simulink model "husky_sim"  (R2019b)
settings: Solver=ode4  StartTime=0.0  StopTime=8  FixedStep=Ts  RelTol=1e-3
InitFcn:
  | init_model;
values from neighbouring files (symbols this model uses):
  backbone_mass_pos_wrt_body = [0.021107, -5.5457e-05, -0.041523]    [func_robot_param.m]
  del_p_FL_1 = [0.0, 0.18, 0.1]    [func_params_ext.m]
  del_p_FL_2 = [0.0, 0, 0.15]    [func_params_ext.m]
  del_y_BL = 0.125/n    (= 0.0125)    [func_params_ext.m]
  del_y_BR = 0.125/n    (= 0.0125)    [func_params_ext.m]
  del_z_BL = z_BL(2:end)-z_BL(1:n)    [func_params_ext.m]
  del_z_BR = z_BR(2:end)-z_BR(1:n)    [func_params_ext.m]
  femur_mass_loc = [2.704e-07, -0.036112, -0.082829]    [func_params_ext.m]    (also in func_robot_param.m)
  hip_orgin_wrt_backbone = [hip_FR_origin_wrt_backbone, hip_FL_origin_wrt_backbone, hip_BR_origin_wrt_backbone, hip_BL_origin_wrt_backbone].'    [func_params_ext.m]    (also in func_robot_param.m)
  leg_params = [l_hip_offset, l1, l2, l3, q_hf_offset, q_hs_offset, q_k_offset]    [func_params_ext.m]
  m = getfield(leg,'mass')    [dynamic_test.m]    (also in pen_init.m = link2.mass; test.mat = 2.2337)
  mu_s = 0.8    [func_params_ext.m]    (also in pen_init.m; test.mat)
  n = 10    [func_params_ext.m]
  p_init = p_init + 1*[0,0,0,  0,0,0,  0,-0,0,   0,0,0]    [func_params_ext.m]
  q_BL_K0 = initial_angle(12)    [func_params_ext.m]
  q_BR_K0 = initial_angle(9)    [func_params_ext.m]
  q_FL_K0 = initial_angle(6)    [func_params_ext.m]
  T_f_back_BL = 0.1/n    (= 0.01)    [func_params_ext.m]
  T_f_back_BR = 0.1/n    (= 0.01)    [func_params_ext.m]
  T_f_FL_1 = 1    [func_params_ext.m]
  T_f_FL_2 = 1    [func_params_ext.m]
  t_start = 0.32    [func_params_ext.m]
  Ts = 0.001    [func_params_ext.m]
  v_y = 0    [func_params_ext.m]
  v_z = 0    [func_params_ext.m]
undefined symbols (not defined in the file or in its folder): body, femur_left, femur_right, hip_left, hip_right, link_left, link_right, tarsus_left, tarsus_right, tibia_left, tibia_right, X, Y, Z
libraries: sm_lib x206, nesl_utility x56, dspsigops x7, Contact_Forces_Lib x4, simulink x2
(part 6 of 6)

== matlab function husky_sim/move_inside_support_triangle ==
  data: q input; del_q_req output; p_leg_end_position_0 output; p_body input; quat_body input; F_n input; F_t input; start_optimizer input; legs_on_ground input; leg_params parameter; backbone_mass_pos_wrt_body parameter; body parameter; hip_orgin_wrt_backbone parameter; femur_left parameter; femur_mass_loc parameter; p_COM_0 output; p_COM_req output; inside_triangle output; mu_s parameter; t_start parameter; t input
% Find change in joint angles necessary to move COM inside support polygon
%
% Inputs: 
%   q - (12x1) all joint angles in the follwoing order
%       [q_FR_HF; q_FR_HS; q_FR_K;
%       q_FL_HF; q_FL_HS; q_FL_K
%       q_BR_HF; q_BR_HS; q_BR_K
%       q_BL_HF; q_BL_HS; q_BL_K]
%   p_body -  (3x1) body positions [x,y,z] relative to world coordinate frame
%   quat_body - (4x1) quaternion repretsentation of body orientation 
%       relative to world coordinate frame
%   F_n: (4x1) normal forces acting on all 4 legs in the following order:
%           FR, FL, BR, BL
%   F_t: (12x1) tangential forces (x,y,z(?)) acting on the 4 legs 
% 
% Prameters: 
%   leg_params - parameters needed for computing FK or IK in each leg
%       [l_hip_offset, l1, l2, l3, q_hf_offset, q_hs_offset, q_k_offset]
%       (see notes)
%   backbone_mass_pos_wrt_body - location [x,y,z] of backbone mass 
%       relative to body cooridnate frame
%   body - structure which contains mass and inertial properties of backbone
%           used to obtain body mass
%   hip_orgin_wrt_backbone - (1x12) position [x,y,z] of hip coordinate frame of
%       each leg relative to body
%   femur_left - structure which contains mass and inertial properties of
%       femur used to obtain mass of femur (same for lef and right femur)
%   femur_mass_loc - (12x1) location [x,y,z] of all 4 femur mass relative to 
%   	hip reference frame
%   mu_s: static coeff of friciton between leg end and ground
%
% Output: 
%   del_q_req - change in joint angles necessary for the COM to be inside
%       cupport polygon, as provided by optimizer
%   p_leg_end_position_0 - (12x1) leg end position relative to world
%       coordinate frame
%   p_COM_0 - current COM position [x,y,z] relative to world coordinate frame
%   p_COM_req - COM position needed to land inside support polygon as
%       computed by optimizer
%   inside_triangle - boolean, 1 if inside support polygon, 0 otherwise
%
% NOTES: 
%   *Currently this only works when 3 legs are on the ground
%   *if optimizer fails or fi currently inside support polygon, 
%           del_q_req returns zeros (12x1)
%   *Currently it is assumed that only three legs (FR, BR, BL) are on the
%   ground if even this might not be true. This is hard coded in
%   TODO: automatically detect which legs are on the ground and compute
%       required correction
%
function [del_q_req, p_leg_end_position_0, p_COM_0, p_COM_req, inside_triangle] =...
    func_move_inside_support_polygon(q, p_body, quat_body, F_n, F_t, start_optimizer, legs_on_ground,...
    leg_params, backbone_mass_pos_wrt_body, body, hip_orgin_wrt_backbone, ...
    femur_left, femur_mass_loc, mu_s, t_start, t)

leg_on_ground_index = find(legs_on_ground);
leg_in1 = (leg_on_ground_index(1)-1)*3*[1 1 1] + [1 2 3];
leg_in2 = (leg_on_ground_index(2)-1)*3*[1 1 1] + [1 2 3];
leg_in3 = (leg_on_ground_index(3)-1)*3*[1 1 1] + [1 2 3];

leg_in = [leg_in1 leg_in2 leg_in3];

leg_out = (find(~legs_on_ground)-1)*3*[1 1 1] + [1 2 3];

% turn quaternion double vector to quaternion array
quaternion_body = quaternion(quat_body.');

% Mass of femur and body
body_mass = body.mass;
femur_mass = femur_left.mass;

p_leg_end_position_0 = func_leg_end_pos(q, p_body, quaternion_body, leg_params, hip_orgin_wrt_backbone);

% Currnet p_COM
p_COM_0 = func_husky_COM(q, p_body, leg_params, femur_mass_loc, body_mass, femur_mass, hip_orgin_wrt_backbone, backbone_mass_pos_wrt_body);
% desiired p_COM
p_COM_des = [p_body(1:2); 0.39];


% Check if inside support polygon
inside_triangle = func_check_inside_polygon(p_COM_0, p_leg_end_position_0, legs_on_ground);

if inside_triangle >= 1 || start_optimizer ~= 1
% if t <= t_start || start_optimizer ~= 1
    p_COM_req = p_COM_0;
    q_req = q;
    del_q_req = q_req - q;
else
    % Find joint cofiguration that moves COM in support polygon
    opts = optimoptions('fmincon','Algorithm','sqp',...
        'OptimalityTolerance',1e-5);
    
%     q_grounded = q([1:2, 7:8, 10:11]);
%     q_swing = q(4:5);
%     q_knee = q([3, 6, 9, 12]);
    q_grounded = q(leg_in);
    q_swing = q(leg_out);
    
    func = @(q_grounded) func_cost(q_grounded, q_swing, p_body, quaternion_body, legs_on_ground, leg_params, femur_mass_loc,...
        body_mass, femur_mass, hip_orgin_wrt_backbone, backbone_mass_pos_wrt_body, p_COM_des, q, p_leg_end_position_0);
    
    x0 = q_grounded;
    
    lb = repmat([-90 -120 -90]*pi/180,1,3);
    ub = repmat([90 120 90]*pi/180,1,3);
    
    nonlcon = @(q_grounded) func_nonlin_cons(q_grounded, q_swing, p_body, quaternion_body, legs_on_ground, F_n, F_t, leg_params, femur_mass_loc,...
    body_mass, femur_mass, hip_orgin_wrt_backbone, backbone_mass_pos_wrt_body, mu_s);
    
    [q_opt_grounded, fval, eflag, output] = fmincon(func,x0,[],[],[],[],...
        lb,ub,nonlcon,opts);
    
    q_opt = [q_opt_grounded(1:3); q_swing; q_opt_grounded(4:end)];
%     q_opt = [q_opt_grounded(1:2); q_knee(1); q_swing(1:2); q_knee(2); q_opt_grounded(3:4); q_knee(3); q_opt_grounded(5:6); q_knee(4)];
    
    % move only if optimizer finds a solution
    if eflag >= 1
        q_req = q_opt;
    else
        % stay in current position
        q_req = q;
    end
    
    del_q_req = q_req - q;
    
    % p_COM location found by optimizer
    p_COM_req = func_husky_COM(q_req, p_body, leg_params, femur_mass_loc, body_mass, femur_mass, hip_orgin_wrt_backbone, backbone_mass_pos_wrt_body);
    
end

end


%======================================================================
% Optimizer

% Cost function
%
% Inputs:
%   q_grounded 
%   q_swing
%   p_body
%   leg_params
%   femur_mass_loc
%   body_mass
%   femur_mass
%   hip_orgin_wrt_backbone
%   backbone_mass_pos_wrt_body
%   p_COM_des
%   q0
%   p_leg_end_position_0
%
% Outputs: J - computed cost
% 
function J = func_cost(q_grounded, q_swing, p_body, quaternion_body, legs_on_ground, leg_params, femur_mass_loc,...
    body_mass, femur_mass, hip_orgin_wrt_backbone, backbone_mass_pos_wrt_body, p_COM_des, q0, p_leg_end_position_0)


leg_on_ground_index = find(legs_on_ground);
leg_float_index = find(~legs_on_ground);

unsorted_matrix = [q_grounded(1:3).', leg_on_ground_index(1);...
                   q_grounded(4:6).', leg_on_ground_index(2);...
                   q_grounded(7:9).', leg_on_ground_index(3);...
                   q_swing.', leg_float_index];
sorted_matrix = sortrows(unsorted_matrix,4);


% q = [q_grounded(1:2); q_knee(1); q_swing(1:2); q_knee(2); q_grounded(3:4); q_knee(3); q_grounded(5:6); q_knee(4)];
% q = [q_grounded(1:3); q_swing; q_grounded(4:end)];
q = [sorted_matrix(1,1:3), sorted_matrix(2,1:3), sorted_matrix(3,1:3), sorted_matrix(4,1:3)].';

p_COM = func_husky_COM(q, p_body, leg_params, femur_mass_loc, body_mass, femur_mass, hip_orgin_wrt_backbone, backbone_mass_pos_wrt_body);

p_leg_end_position = func_leg_end_pos(q, p_body, quaternion_body, leg_params, hip_orgin_wrt_backbone);

J = 1e3*norm(p_COM(1:3) - p_COM_des(1:3))^2 + 1e4*norm(q - q0)^2;

% 1e4*norm(p_leg_end_position([3,9,12]) - p_leg_end_position_0([3,9,12]))^2;

end

% Nonlinear Constraints
%
% Inputs:
%   q_grounded 
%   q_swing
%   p_body
%   quaternion_body
%   F_n
%   F_t
%   leg_params
%   femur_mass_loc
%   body_mass
%   femur_mass
%   hip_orgin_wrt_backbone
%   backbone_mass_pos_wrt_body
%   mu_s
%
% Outputs: [c, ceq]
%   c - inequality constraints
%       * Ensure x,y components of p_COM is within support polygon
%       * Make sure the grounded legs do not move by satisfying 
%           normal force > 0
%           |tangnetial force| < mu_static*|normal force|
%
%   ceq - equality constraints (none)
% 
function [c, ceq] = func_nonlin_cons(q_grounded, q_swing, p_body, quaternion_body, legs_on_ground, F_n, F_t, leg_params, femur_mass_loc,...
    body_mass, femur_mass, hip_orgin_wrt_backbone, backbone_mass_pos_wrt_body, mu_s)

c = zeros(1,3);
ceq = 0;

leg_on_ground_index = find(legs_on_ground);
leg_float_index = find(~legs_on_ground);

unsorted_matrix = [q_grounded(1:3).', leg_on_ground_index(1);...
                   q_grounded(4:6).', leg_on_ground_index(2);...
                   q_grounded(7:9).', leg_on_ground_index(3);...
                   q_swing.', leg_float_index];
sorted_matrix = sortrows(unsorted_matrix,4);

% q_swing: leg in air is fixed, not perturbed by optimizer
% q = [q_grounded(1:2); q_knee(1); q_swing(1:2); q_knee(2); q_grounded(3:4); q_knee(3); q_grounded(5:6); q_knee(4)];
% q = [q_grounded(1:3); q_swing; q_grounded(4:end)];
q = [sorted_matrix(1,1:3), sorted_matrix(2,1:3), sorted_matrix(3,1:3), sorted_matrix(4,1:3)].';

% Seperate tangential and normal forces 
F_n_BR = F_n(3);
F_n_BL = F_n(4);
F_t_BR = F_t([7,8]);
F_t_BL = F_t([10,11]);

p_leg_end_position_abs = func_leg_end_pos(q, p_body, quaternion_body, leg_params, hip_orgin_wrt_backbone);

% Reduce size of triangle
del_pos = 0.02; % in meter

p_leg_end_position_rel = p_leg_end_position_abs - repmat(p_body,4,1);
% reduce the sides of the triangle by del_pos meters
p_leg_end_position_adjusted = p_leg_end_position_abs - sign(p_leg_end_position_rel)*del_pos;

p_COM = func_husky_COM(q, p_body, leg_params, femur_mass_loc, body_mass, femur_mass, hip_orgin_wrt_backbone, backbone_mass_pos_wrt_body);

[~, s, t] = func_check_inside_polygon(p_COM, p_leg_end_position_adjusted, legs_on_ground);

% p_COM inside triangle when s >=0, t>=0 and s + t <= 1
% inequality defined only for c <= 0, so changing signs
%
% Note adding slack variable alpha to constraint so COM doesn't 
% sit at the edge of support polygon
alpha = 0.04;
c(1) = -(s - alpha);
c(2) = -(t - alpha);
c(3) = s + t - 1 + alpha;
% c(4:5) = -[F_n_BR; F_n_BL];
% c(6:7) = abs(F_t_BR) - mu_s*abs(F_n_BR);
% c(8:9) = abs(F_t_BL) - mu_s*abs(F_n_BL);

% c(4:12) = abs(p_leg_end_position([1:3, 7:12]) - p_leg_end_position_0([1:3, 7:12])) - 0.01;

end

%======================================================================
% Check if currently inside support polygon
%
% Inputs: 
%   p_COM - current COM position [x,y,z]
%   p_leg_end_position - (12x1) leg end position relative to world
%       coordinate frame
%
% OutputsL
%   inside_triangle - boolean, 1 if inside support polygon, 0 otherwise
%   [s, t] - variables used in Barycentric coordinates to determine if
%       point inside a 2D triangle, will be used to determine if COM inside
%       support polygon
%
% NOTES: 
%
function [inside_triangle, s, t] = func_check_inside_polygon(p_COM, p_leg_end_position, legs_on_ground)

leg_on_ground_index = find(legs_on_ground);

leg_1_indx = (leg_on_ground_index(1)-1)*3*[1 1 1] + [1 2 3];
leg_2_indx = (leg_on_ground_index(2)-1)*3*[1 1 1] + [1 2 3];
leg_3_indx = (leg_on_ground_index(3)-1)*3*[1 1 1] + [1 2 3];

% Individual feet end poisitions
p_1 = p_leg_end_position(leg_1_indx);
p_2 = p_leg_end_position(leg_2_indx);
p_3 = p_leg_end_position(leg_3_indx);

% points/vertices of triangle
A = p_1(1:2); B = p_2(1:2); C = p_3(1:2);

% The equation for a point in Bary centric coordinate is defined as:
% p = A + (B - A)*s + (C - A)*t;
%   where A,B,B are three points of a triangle
% The point p is inside the triangle if 0 < s, t < 1 and s+t<1

% Computing s and t will help determine

v0 = B - A; v1 = C - A; v2 = p_COM(1:2) - A;

% Compute dot products
v0v0 = dot(v0, v0);
v0v1 = dot(v0, v1);
v1v0 = dot(v1, v0);
v1v1 = dot(v1, v1);
v2v1 = dot(v2, v1);
v2v0 = dot(v2, v0);

% Compute barycentric coordinates
LHS = [v0v0 v1v0; v0v1 v1v1];
temp = LHS\[v2v0; v2v1];
s = temp(1);
t = temp(2);

% Alternative approach to computing as and t
% invDenom = 1/(v0v0 * v1v1 - v0v1 * v0v1);
% s = (v1v1*v2v0 - v0v1*v2v1)*invDenom;
% t = (v0v0*v2v1 - v0v1*v2v0)*invDenom;

% returns 1 if in triangle
inside_triangle = double((s >= 0) && (t >= 0) && (s + t <= 1));

end



%======================================================================
% COM and leg end position

% Find position of COM wrt world coordinate frame
function p_COM = func_husky_COM(q, p_body, leg_params, femur_mass_loc, body_mass, femur_mass, hip_orgin_wrt_backbone, backbone_mass_pos_wrt_body)

% COM position of femur
p_femur_COM_wrt_hip = func_femur_COM(q, leg_params, femur_mass_loc);
p_femur_COM = p_femur_COM_wrt_hip + hip_orgin_wrt_backbone;
p_femur_COM_FR = p_femur_COM(1:3);
p_femur_COM_FL = p_femur_COM(4:6);
p_femur_COM_BR = p_femur_COM(7:9);
p_femur_COM_BL = p_femur_COM(10:12);

p_COM_wrt_body = (body_mass*backbone_mass_pos_wrt_body.' + femur_mass*p_femur_COM_FR + ...
    femur_mass*p_femur_COM_FL + femur_mass*p_femur_COM_BR + femur_mass*p_femur_COM_BL)/(body_mass + 4*femur_mass);

p_COM = p_COM_wrt_body + p_body;

end

function p_leg_end_position = func_leg_end_pos(q, p_body, quaternion_body, leg_params, hip_orgin_wrt_backbone)

% Get leg end position relative to hip, based on FK
p_end_wrt_hip = func_husky_FK(q, leg_params);

% feet end relative to body ref frame
p_end_wrt_body = hip_orgin_wrt_backbone + p_end_wrt_hip;

% apply rotation to feet end based on rotation of body ref frame
p_FR_end_wrt_body_rotated = rotatepoint(quaternion_body, p_end_wrt_body(1:3).').';
p_FL_end_wrt_body_rotated = rotatepoint(quaternion_body, p_end_wrt_body(4:6).').';
p_BR_end_wrt_body_rotated = rotatepoint(quaternion_body, p_end_wrt_body(7:9).').';
p_BL_end_wrt_body_rotated = rotatepoint(quaternion_body, p_end_wrt_body(10:12).').';

p_end_wrt_body_rotated = [p_FR_end_wrt_body_rotated; p_FL_end_wrt_body_rotated; p_BR_end_wrt_body_rotated; p_BL_end_wrt_body_rotated];

% feet end location relaitve to world coordinate frame
p_leg_end_position = repmat(p_body,4,1) + p_end_wrt_body_rotated;

end


%======================================================================
% Forward Kinmeatics

% Find current leg end position based on encoder readings (in rads)
%
function p_end_req = func_husky_FK(q_curr, leg_params)

q_curr_FR = q_curr(1:3);
q_curr_FL = q_curr(4:6);
q_curr_BR = q_curr(7:9);
q_curr_BL = q_curr(10:12);

p_end_FR_curr = func_FK_right(q_curr_FR,leg_params);
p_end_FL_curr = func_FK_left(q_curr_FL,leg_params);
p_end_BR_curr = func_FK_right(q_curr_BR,leg_params);
p_end_BL_curr = func_FK_left(q_curr_BL,leg_params);

p_end_req = [p_end_FR_curr; p_end_FL_curr; p_end_BR_curr; p_end_BL_curr];

end

function p_end = func_FK_right(q,leg_param)
%FUNC_FK
%    P_END = FUNC_FK(IN1,IN2)

%    This function was generated by the Symbolic Math Toolbox version 8.3.
%    12-Dec-2019 10:24:24

% Right leg FK
% Obtain feet end position [x, y, z] based on leg angles [q_hf, q_hs, q_k]
%
% Inputs: q = [q_hf, q_hs, q_k]; hip frontal, hip sagittal and knee angles
%         leg_params = [l_offset l1 l2 l3] leg lengths (see notes)
%
% Output: p_end = [x; y; z] coordinates of feet end
% by Pravin Dangol, Boston, MA
l1 = leg_param(2);
l2 = leg_param(3);
l3 = leg_param(4);
l_offset = leg_param(1);
q_hf = q(1);
q_hs = q(2);
q_k = q(3);
q_hf_offset = leg_param(5);
q_hs_offset = leg_param(6);
q_k_offset = leg_param(7);
p_end = [-l2.*sin(q_hs+q_k+q_hs_offset+q_k_offset)+l1.*sin(q_hs+q_hs_offset)+l3.*sin(q_hs+q_hs_offset);...
    l_offset.*sin(q_hf-q_hf_offset)-l1.*cos(q_hf-q_hf_offset).*cos(q_hs+q_hs_offset)-l3.*cos(q_hf-q_hf_offset).*cos(q_hs+q_hs_offset)+l2.*cos(q_hf-q_hf_offset).*cos(q_hs+q_hs_offset).*cos(q_k+q_k_offset)-l2.*cos(q_hf-q_hf_offset).*sin(q_hs+q_hs_offset).*sin(q_k+q_k_offset);...
    l_offset.*cos(q_hf-q_hf_offset)+l1.*sin(q_hf-q_hf_offset).*cos(q_hs+q_hs_offset)+l3.*sin(q_hf-q_hf_offset).*cos(q_hs+q_hs_offset)-l2.*sin(q_hf-q_hf_offset).*cos(q_hs+q_hs_offset).*cos(q_k+q_k_offset)+l2.*sin(q_hf-q_hf_offset).*sin(q_hs+q_hs_offset).*sin(q_k+q_k_offset)];

% p_end = reshape(p_end,1,12);

end

function p_end = func_FK_left(q,leg_param)
%FUNC_FK_LEFT
%    P_END = FUNC_FK_LEFT(IN1,IN2)

%    This function was generated by the Symbolic Math Toolbox version 8.3.
%    12-Dec-2019 10:24:24

% Left leg FK
% Obtain feet end position [x, y, z] based on leg angles [q_hf, q_hs, q_k]
%
% Inputs: q = [q_hf, q_hs, q_k]; hip frontal, hip sagittal and knee angles
%         leg_params = [l_offset l1 l2 l3] leg lengths (see notes)
%
% Output: p_end = [x; y; z] coordinates of feet end
% by Pravin Dangol, Boston, MA
l1 = leg_param(2);
l2 = leg_param(3);
l3 = leg_param(4);
l_offset = leg_param(1);
q_hf = q(1);
q_hs = q(2);
q_k = q(3);
q_hf_offset = leg_param(5);
q_hs_offset = leg_param(6);
q_k_offset = leg_param(7);
p_end = [-l2.*sin(q_hs+q_k+q_hs_offset+q_k_offset)+l1.*sin(q_hs+q_hs_offset)+l3.*sin(q_hs+q_hs_offset);...
    -l_offset.*sin(q_hf-q_hf_offset)+l1.*cos(q_hf-q_hf_offset).*cos(q_hs+q_hs_offset)+l3.*cos(q_hf-q_hf_offset).*cos(q_hs+q_hs_offset)-l2.*cos(q_hf-q_hf_offset).*cos(q_hs+q_hs_offset).*cos(q_k+q_k_offset)+l2.*cos(q_hf-q_hf_offset).*sin(q_hs+q_hs_offset).*sin(q_k+q_k_offset);...
    l_offset.*cos(q_hf-q_hf_offset)+l1.*sin(q_hf-q_hf_offset).*cos(q_hs+q_hs_offset)+l3.*sin(q_hf-q_hf_offset).*cos(q_hs+q_hs_offset)-l2.*sin(q_hf-q_hf_offset).*cos(q_hs+q_hs_offset).*cos(q_k+q_k_offset)+l2.*sin(q_hf-q_hf_offset).*sin(q_hs+q_hs_offset).*sin(q_k+q_k_offset)];

end

%======================================================================
% COM location

% Find femur COM position based on encoder readings (in rads)
%
function p_femur_COM_wrt_hip = func_femur_COM(q_curr, leg_params,femur_mass_pos)

q_curr_FR = q_curr(1:3);
q_curr_FL = q_curr(4:6);
q_curr_BR = q_curr(7:9);
q_curr_BL = q_curr(10:12);

p_femur_COM_FR = func_femur_COM_right(q_curr_FR,leg_params,femur_mass_pos);
p_femur_COM_FL = func_femur_COM_left(q_curr_FL,leg_params,femur_mass_pos);
p_femur_COM_BR = func_femur_COM_right(q_curr_BR,leg_params,femur_mass_pos);
p_femur_COM_BL = func_femur_COM_left(q_curr_BL,leg_params,femur_mass_pos);

p_femur_COM_wrt_hip = [p_femur_COM_FR; p_femur_COM_FL; p_femur_COM_BR; p_femur_COM_BL];

end

function p_femur_COM = func_femur_COM_right(q,leg_params,femur_mass_pos)
%FUNC_FEMUR_COM_RIGHT
%    p_femur_COM = FUNC_FEMUR_COM_RIGHT(IN1,IN2,IN3)

%    This function was generated by the Symbolic Math Toolbox version 8.4.
%    08-Jan-2020 22:02:50

% Right leg HS COM location
% Obtain COM position [x, y, z] of femur based on leg angles [q_hf, q_hs, q_k]
%
% Inputs: q = [q_hf, q_hs, q_k]; hip frontal, hip sagittal and knee angles
%         leg_params = [l_offset l1 l2 l3] leg lengths (see notes)
%         femur_mass_pos = [x y z] position of femur COM reltiave to femur base ref frame
%
% Output: p_end = [x; y; z] coordinates of feet end
% by Pravin Dangol, Boston, MA
l_offset = leg_params(1);
m_femur_x = femur_mass_pos(1);
m_femur_y = femur_mass_pos(2);
m_femur_z = femur_mass_pos(3);
q_hf = q(1);
q_hs = q(2);
q_hf_offset = leg_params(5);
q_hs_offset = leg_params(6);
p_femur_COM = [m_femur_x.*cos(q_hs+q_hs_offset)-m_femur_z.*sin(q_hs+q_hs_offset);...
    l_offset.*sin(q_hf-q_hf_offset)-m_femur_y.*sin(q_hf-q_hf_offset)+m_femur_z.*cos(q_hf-q_hf_offset).*cos(q_hs+q_hs_offset)+m_femur_x.*cos(q_hf-q_hf_offset).*sin(q_hs+q_hs_offset);...
    l_offset.*cos(q_hf-q_hf_offset)-m_femur_y.*cos(q_hf-q_hf_offset)-m_femur_z.*sin(q_hf-q_hf_offset).*cos(q_hs+q_hs_offset)-m_femur_x.*sin(q_hf-q_hf_offset).*sin(q_hs+q_hs_offset)];

end

function p_femur_COM = func_femur_COM_left(q,leg_params,femur_mass_pos)
%FUNC_FEMUR_COM_LEFT
%    p_femur_COM = FUNC_FEMUR_COM_LEFT(IN1,IN2,IN3)

%    This function was generated by the Symbolic Math Toolbox version 8.4.
%    08-Jan-2020 22:02:58

% Left leg HS COM location
% Obtain COM position [x, y, z] of femur based on leg angles [q_hf, q_hs, q_k]
%
% Inputs: q = [q_hf, q_hs, q_k]; hip frontal, hip sagittal and knee angles
%         leg_params = [l_offset l1 l2 l3] leg lengths (see notes)
%         femur_mass_pos = [x y z] position of femur COM reltiave to femur base ref frame
%
% Output: p_end = [x; y; z] coordinates of feet end
% by Pravin Dangol, Boston, MA
l_offset = leg_params(1);
m_femur_x = femur_mass_pos(1);
m_femur_y = femur_mass_pos(2);
m_femur_z = femur_mass_pos(3);
q_hf = q(1);
q_hs = q(2);
q_hf_offset = leg_params(5);
q_hs_offset = leg_params(6);
p_femur_COM = [m_femur_x.*cos(q_hs+q_hs_offset)-m_femur_z.*sin(q_hs+q_hs_offset);...
    -l_offset.*sin(q_hf-q_hf_offset)+m_femur_y.*sin(q_hf-q_hf_offset)-m_femur_z.*cos(q_hf-q_hf_offset).*cos(q_hs+q_hs_offset)-m_femur_x.*cos(q_hf-q_hf_offset).*sin(q_hs+q_hs_offset);...
    l_offset.*cos(q_hf-q_hf_offset)+m_femur_y.*cos(q_hf-q_hf_offset)-m_femur_z.*sin(q_hf-q_hf_offset).*cos(q_hs+q_hs_offset)-m_femur_x.*sin(q_hf-q_hf_offset).*sin(q_hs+q_hs_offset)];

end

== matlab function husky_sim/Foot placement/MATLAB Function ==
  data: impact input; pair1_on_ground output; pair2_on_ground output
function [pair1_on_ground, pair2_on_ground] = func_leg_contact(impact)

if impact([1,4]) == 1
    pair1_on_ground = 1;
else
    pair1_on_ground = 0;
end

if impact([2,3]) == 1
    pair2_on_ground = 1;
else
    pair2_on_ground = 0;
end

end

== stateflow chart husky_sim/Foot placement/Chart ==
  state Phase2
    entry:
    del_pf = [0,0,0, 0,0,z_max,...
    0,0,z_max,  0,0,0];
  state Start
  state Phase1
    entry:
    del_pf = [0,0,z_max, 0,0,0,...
    0,0,0,  0,0,z_max];
  state Phase3
    entry:
    del_pf = [0,0,0, 0,0,0,...
    0,0,0,  0,0,0];
  Phase1 -> Phase2 [order 1] : [pair2_on_ground==1]
  Start -> Phase1 : [pair1_on_ground==1]
  (default) -> Start
  Phase2 -> Phase1 [order 1] : [pair1_on_ground==1]
  Phase1 -> Phase3 [order 2] : [start==0]
  Phase2 -> Phase3 [order 2] : [start==0]
  data: pair1_on_ground input; pair2_on_ground input; start input; z_max input; del_pf output

== matlab function husky_sim/Foot placement/husky_IK ==
  data: p_des input; q_des output; p_hf input; leg_params parameter
% Obtain leg angles [q_hf, q_hs, q_k] (in rads) from desired feet end  
%   cartesian coordinates for one leg
%
% Inputs: p_end_des = [x_des; y_des; z_des] desired coordinates of feet end 
%           reative to reference frame (located at frontal hip motor)
%         p_hf = [x0; y0; z0] body reference frame at hip frontal motor
%         leg_params = [l_offset l1 l2 l3,...
%           q_hf_offset q_hs_offset q_k_offset] leg lengths and angle
%           offsets (in rads) - see notes
% 
% Prameters: 
%   leg_params - parameters needed for computing FK or IK in each leg
%       [l_hip_offset, l1, l2, l3, q_hf_offset, q_hs_offset, q_k_offset]
%       (see notes)
%
% Output: q_des =  (12x1)[q_HF, q_HS, q_K] hip frontal, hip sagittal and knee
%  angles (in rads) based on IK in the following order
%       [q_FR_HF; q_FR_HS; q_FR_K;
%       q_FL_HF; q_FL_HS; q_FL_K
%       q_BR_HF; q_BR_HS; q_BR_K
%       q_BL_HF; q_BL_HS; q_BL_K]
%
% NOTES: 
%
% by Pravin Dangol, Boston, MA, 12-05-19
function q_des = func_IK_Husky(p_des, p_hf, leg_params)

p_hf_FR = p_hf(1:3);
p_hf_FL = p_hf(4:6);
p_hf_BR = p_hf(7:9);
p_hf_BL = p_hf(10:12);

p_des_FR = p_des(1:3);
p_des_FL = p_des(4:6);
p_des_BR = p_des(7:9);
p_des_BL = p_des(10:12);


q_FR_des = func_IK_right_leg(p_des_FR, p_hf_FR, leg_params);

q_BR_des = func_IK_right_leg(p_des_BR, p_hf_BR, leg_params);

% Left leg IK, different function used to stay consistent with chosen 
% sign convention, i.e. positive q_hf is leg rotating outwards, which is
% coutner clockwise, as apposed to clockwise for right legs
q_FL_des = func_IK_left_leg(p_des_FL, p_hf_FL, leg_params);

q_BL_des = func_IK_left_leg(p_des_BL, p_hf_BL, leg_params);


q_des = [q_FR_des; q_FL_des; q_BR_des; q_BL_des];


end

% inverse kinematics
function qd = func_IK_right_leg(p_des, p_hf, leg_params)

l_offset = leg_params(1);
l1 = leg_params(2);
l2 = leg_params(3);
l3 = leg_params(4);
q_hf_offset = leg_params(5);
q_hs_offset  = leg_params(6);
q_k_offset = leg_params(7);

% Length and parameters from the 2D leg plane, see notes
k = l1/l3;
l5 = l_offset;
l9 = sqrt((p_des(1)-p_hf(1))^2);
l6 = sqrt((p_des(3)-p_hf(3))^2+(p_des(2)-p_hf(2))^2);

% saturate lowest values to 0 before passing to sqrt()
l6_l5 = max(l6^2-l5^2,0);

l8 = sqrt(l6_l5);
lv = sqrt(l9^2+l8^2);
lv2 = lv/(k+1);
% lv1 = lv2*k;
l2a = l2/(k+1);
% l2b = l2a*k;

% Values from triangle ABC formed by the feet end, hip frontal and hip
% sagittal (see notes)
[~,q_k_prime,~] = func_triangle_angles(l2a,lv2,l3);

% calculate q_hf
beta2 = atan2(l8,l5);
temp2 = -(p_des(2)-p_hf(2))/sqrt(l5^2+l8^2);

% Saturate inputs to asin, so there is no complex output
temp2 = min(max(temp2, -1), 1);

q_hf_prime = pi-asin(temp2)-beta2;

% Note: need to keep q_hf_prime within 0 and pi inorder to avoid 1/0
%   Add saturation below

% calculate q_hs
l8_actual =  -(l5*cos(q_hf_prime) + (p_des(3)-p_hf(3)))/(sin(q_hf_prime));
% l8_actual = -(l5*cos(q_hf_prime) + (p_des(3)-p_hf(3)))/(sin(q_hf_prime));
l9_actual = (p_des(1)-p_hf(1));
beta1 = atan2(l8_actual,l9_actual);
temp1 = ((l1+l3)-l2*cos(q_k_prime))/sqrt(l8_actual^2+l9_actual^2);

% Saturate inputs to asin, so there is no complex output
temp1 = min(max(temp1, -1), 1);

q_hs_prime = pi-asin(temp1)-beta1;


% Subtract offsets from angles so 0 angle corresponds with the zero/startup 
%  configuration of husky
q_hf = q_hf_offset - q_hf_prime ;
q_hs = q_hs_prime - q_hs_offset;
q_k = q_k_prime - q_k_offset;

qd = [q_hf; q_hs; q_k];

end

function qd = func_IK_left_leg(p_des, p_hf, leg_params)

l_offset = -leg_params(1);
l1 = leg_params(2);
l2 = leg_params(3);
l3 = leg_params(4);
q_hf_offset = leg_params(5);
q_hs_offset  = leg_params(6);
q_k_offset = leg_params(7);

% Length and parameters from the 2D leg plane, see notes
k = l1/l3;
l5 = l_offset;
l9 = sqrt((p_des(1)-p_hf(1))^2);
l6 = sqrt((p_des(3)-p_hf(3))^2+(p_des(2)-p_hf(2))^2);

% saturate lowest values to 0 before passing to sqrt()
l6_l5 = max(l6^2-l5^2,0);

l8 = sqrt(l6_l5);
lv = sqrt(l9^2+l8^2);
lv2 = lv/(k+1);
% lv1 = lv2*k;
l2a = l2/(k+1);
% l2b = l2a*k;

% Values from triangle ABC formed by the feet end, hip frontal and hip
% sagittal (see notes)
[~,q_k_prime,~] = func_triangle_angles(l2a,lv2,l3);

% calculate q_hf
beta2 = atan2(l8,l5);
temp2 = -(p_des(2)-p_hf(2))/sqrt(l5^2+l8^2);

% Saturate inputs to asin, so there is no complex output
temp2 = min(max(temp2, -1), 1);

q_hf_prime = pi-asin(temp2)-beta2;

% Note: need to keep q_hf_prime within 0 and pi inorder to avoid 1/0
%   Add saturation below

% calculate q_hs
l8_actual =  -(l5*cos(q_hf_prime) + (p_des(3)-p_hf(3)))/(sin(q_hf_prime));
% l8_actual = -(l5*cos(q_hf_prime) + (p_des(3)-p_hf(3)))/(sin(q_hf_prime));
l9_actual = (p_des(1)-p_hf(1));
beta1 = atan2(l8_actual,l9_actual);
temp1 = ((l1+l3)-l2*cos(q_k_prime))/sqrt(l8_actual^2+l9_actual^2);

% Saturate inputs to asin, so there is no complex output
temp1 = min(max(temp1, -1), 1);

q_hs_prime = pi-asin(temp1)-beta1;


% Subtract offsets from angles so 0 angle corresponds with the zero/startup 
%  configuration of husky
q_hf = q_hf_offset - q_hf_prime ;
q_hs = q_hs_prime - q_hs_offset;
q_k = q_k_prime - q_k_offset;

% NOTE: q_hf should be negative due to change in sign convention for leg leg,
% compared to right
qd = [-q_hf; q_hs; q_k];


end

% use trigonometry to obtain the angles of a triangle 
%
% input:
%   lines with dims a,b and c
%
% output:
%   theta1: angle between a and c
%   theta2: angle between c and b
%   theta3: angle between b and a
%
% By Xuyang Sun
function [theta1,theta2,theta3] = func_triangle_angles(a,b,c)
c1 = func_law_of_cosine(a,b,c);
c2 = func_law_of_cosine(b,a,c);
c3 = func_law_of_cosine(c,b,a);

% Saturate inputs to acos, so there is no complex output
c1 = min(max(c1, -1), 1);
c2 = min(max(c2, -1), 1);
c3 = min(max(c3, -1), 1);

theta1 = acos(c1);
theta2 = acos(c2);
theta3 = acos(c3);
end


% obtain cos(theta) based on given the lengths of a triangle
%
% input:
%   C: dim of line in front of theta
%   A, B: dim of lines adjacent to theta
%
% output:
%   q: cos(theta)
%
% By Xuyang Sun
function q = func_law_of_cosine(C,A,B)

% if A == 0 || B == 0
%     
% end

q = (-C^2+A^2+B^2)/(2*A*B);

end

== matlab function husky_sim/Foot placement/cubic_traj_waypoints ==
  data: t input; p_end_des output; p0 input; pf input; v0 input; vf input; T_f input
function p_end_des = func_cubic_trajectory(t, p0, pf, v0, vf, T_f)

p0_FR = p0(1:3);
p0_FL = p0(4:6);
p0_BR = p0(7:9);
p0_BL = p0(10:12);

pf_FR = pf(1:3);
pf_FL = pf(4:6);
pf_BR = pf(7:9);
pf_BL = pf(10:12);

v0_FR = v0(1:3);
v0_FL = v0(4:6);
v0_BR = v0(7:9);
v0_BL = v0(10:12);

vf_FR = vf(1:3);
vf_FL = vf(4:6);
vf_BR = vf(7:9);
vf_BL = vf(10:12);

% NOTE: currently all legs must have same time to desired position
%
% Need to change this later so legs can move independently
T_f_FR = T_f(1);
T_f_FL = T_f(1);
T_f_BR = T_f(1);
T_f_BL = T_f(1);



[a0_FR,a1_FR,a2_FR,a3_FR] = func_cubic_traj_coeff(p0_FR,pf_FR,v0_FR,vf_FR, T_f_FR);

[a0_FL,a1_FL,a2_FL,a3_FL] = func_cubic_traj_coeff(p0_FL,pf_FL,v0_FL,vf_FL, T_f_FL);

[a0_BR,a1_BR,a2_BR,a3_BR] = func_cubic_traj_coeff(p0_BR,pf_BR,v0_BR,vf_BR, T_f_BR);

[a0_BL,a1_BL,a2_BL,a3_BL] = func_cubic_traj_coeff(p0_BL,pf_BL,v0_BL,vf_BL, T_f_BL);


p_end_FR = a0_FR + a1_FR.*t + a2_FR.*t^2 + a3_FR.*t^3;
p_end_FL = a0_FL + a1_FL.*t + a2_FL.*t^2 + a3_FL.*t^3;
p_end_BR = a0_BR + a1_BR.*t + a2_BR.*t^2 + a3_BR.*t^3;
p_end_BL = a0_BL + a1_BL.*t + a2_BL.*t^2 + a3_BL.*t^3;

p_end_des = [p_end_FR; p_end_FL; p_end_BR; p_end_BL];

end





% coeffs for x y z axis for 1 leg
function [a0,a1,a2,a3] = func_cubic_traj_coeff(p0,pf,v0,vf, T_f)

x0 = p0(1);
xf = pf(1);
dx0 = v0(1);
dxf = vf(1);

y0 = p0(2);
yf = pf(2);
dy0 = v0(2);
dyf = vf(2);

z0 = p0(3);
zf = pf(3);
dz0 = v0(3);
dzf = vf(3);

% Generate coefficients for cubic position trajectory in the form:
%   p = a0 + a1*t + a2*t^2 + a3*t^3
% Resulting in velocity trajectory:
%   dp = a1 + 2*a2*t + 3*a3*t^2

[a0x,a1x,a2x,a3x] = get_coeff(x0,xf,dx0,dxf, T_f);

[a0y,a1y,a2y,a3y] = get_coeff(y0,yf,dy0,dyf, T_f);

[a0z,a1z,a2z,a3z] = get_coeff(z0,zf,dz0,dzf, T_f);

a0 = [a0x; a0y; a0z];
a1 = [a1x; a1y; a1z];
a2 = [a2x; a2y; a2z];
a3 = [a3x; a3y; a3z];

end

% Generate coefficients for cubic trajectory in the form:
%   p = a0 + a1*t + a2*t^2 + a3*t^3
%   dp = a1 + 2*a2*t + 3*a3*t^2
function [a0,a1,a2,a3] = get_coeff(p0,pf,v0,vf, T_f)

a0 = p0;
a1 = v0;

A = [T_f^2 T_f^3; 2*T_f 3*T_f^2];

B = [pf - a0 - a1*T_f; vf - a1];

temp = A\B;

a2 = temp(1);
a3 = temp(2);

end

== matlab function husky_sim/Foot placement/husky_FK ==
  data: q_curr input; p_end_req output double size=[12,1]; leg_params parameter
% Find current leg end position based on encoder readings (in reads)
%
% Inputs: 
%   q_curr - (12x1) current joint angles in the following order
%       [q_FR_HF; q_FR_HS; q_FR_K;
%       q_FL_HF; q_FL_HS; q_FL_K
%       q_BR_HF; q_BR_HS; q_BR_K
%       q_BL_HF; q_BL_HS; q_BL_K]
% 
% Prameters: 
%   leg_params - parameters needed for computing FK or IK in each leg
%       [l_hip_offset, l1, l2, l3, q_hf_offset, q_hs_offset, q_k_offset]
%       (see notes)
%   backbone_mass_pos_wrt_body - location [x,y,z] of backbone mass 
%       relative to body cooridnate frame
%   body - structure which contains mass and inertial properties of backbone
%           used to obtain body mass
%   hip_orgin_wrt_backbone - (1x12) position [x,y,z] of hip coordinate frame of
%       each leg relative to body
%   femur_left - structure which contains mass and inertial properties of
%       femur used to obtain mass of femur (same for lef and right femur)
%   femur_mass_loc - (12x1) location [x,y,z] of all 4 femur mass relative to 
%   	hip reference frame
%
% Output: 
%   p_end_req - (12x1) feet end positions [FR, FL, BR, BL] relative to 
%           respsective leg hip coordinate frame
%
% NOTES: 
%
% By Pravin Dangol, 12-05-19 (approx), Boston, MA
function p_end_req = func_husky_FK(q_curr, leg_params)

q_curr_FR = q_curr(1:3);
q_curr_FL = q_curr(4:6);
q_curr_BR = q_curr(7:9);
q_curr_BL = q_curr(10:12);

p_end_FR_curr = func_FK_right(q_curr_FR,leg_params);
p_end_FL_curr = func_FK_left(q_curr_FL,leg_params);
p_end_BR_curr = func_FK_right(q_curr_BR,leg_params);
p_end_BL_curr = func_FK_left(q_curr_BL,leg_params);

p_end_req = [p_end_FR_curr; p_end_FL_curr; p_end_BR_curr; p_end_BL_curr];

end

function p_end = func_FK_right(q,leg_param)
%FUNC_FK
%    P_END = FUNC_FK(IN1,IN2)

%    This function was generated by the Symbolic Math Toolbox version 8.3.
%    12-Dec-2019 10:24:24

% Right leg FK
% Obtain feet end position [x, y, z] based on leg angles [q_hf, q_hs, q_k]
%
% Inputs: q = [q_hf, q_hs, q_k]; hip frontal, hip sagittal and knee angles
%         leg_params = [l_offset l1 l2 l3] leg lengths (see notes)
%
% Output: p_end = [x; y; z] coordinates of feet end
% by Pravin Dangol, Boston, MA
l1 = leg_param(2);
l2 = leg_param(3);
l3 = leg_param(4);
l_offset = leg_param(1);
q_hf = q(1);
q_hs = q(2);
q_k = q(3);
q_hf_offset = leg_param(5);
q_hs_offset = leg_param(6);
q_k_offset = leg_param(7);
p_end = [-l2.*sin(q_hs+q_k+q_hs_offset+q_k_offset)+l1.*sin(q_hs+q_hs_offset)+l3.*sin(q_hs+q_hs_offset);...
    l_offset.*sin(q_hf-q_hf_offset)-l1.*cos(q_hf-q_hf_offset).*cos(q_hs+q_hs_offset)-l3.*cos(q_hf-q_hf_offset).*cos(q_hs+q_hs_offset)+l2.*cos(q_hf-q_hf_offset).*cos(q_hs+q_hs_offset).*cos(q_k+q_k_offset)-l2.*cos(q_hf-q_hf_offset).*sin(q_hs+q_hs_offset).*sin(q_k+q_k_offset);...
    l_offset.*cos(q_hf-q_hf_offset)+l1.*sin(q_hf-q_hf_offset).*cos(q_hs+q_hs_offset)+l3.*sin(q_hf-q_hf_offset).*cos(q_hs+q_hs_offset)-l2.*sin(q_hf-q_hf_offset).*cos(q_hs+q_hs_offset).*cos(q_k+q_k_offset)+l2.*sin(q_hf-q_hf_offset).*sin(q_hs+q_hs_offset).*sin(q_k+q_k_offset)];

% p_end = reshape(p_end,1,12);

end

function p_end = func_FK_left(q,leg_param)
%FUNC_FK_LEFT
%    P_END = FUNC_FK_LEFT(IN1,IN2)

%    This function was generated by the Symbolic Math Toolbox version 8.3.
%    12-Dec-2019 10:24:24

% Left leg FK
% Obtain feet end position [x, y, z] based on leg angles [q_hf, q_hs, q_k]
%
% Inputs: q = [q_hf, q_hs, q_k]; hip frontal, hip sagittal and knee angles
%         leg_params = [l_offset l1 l2 l3] leg lengths (see notes)
%
% Output: p_end = [x; y; z] coordinates of feet end
% by Pravin Dangol, Boston, MA
l1 = leg_param(2);
l2 = leg_param(3);
l3 = leg_param(4);
l_offset = leg_param(1);
q_hf = q(1);
q_hs = q(2);
q_k = q(3);
q_hf_offset = leg_param(5);
q_hs_offset = leg_param(6);
q_k_offset = leg_param(7);
p_end = [-l2.*sin(q_hs+q_k+q_hs_offset+q_k_offset)+l1.*sin(q_hs+q_hs_offset)+l3.*sin(q_hs+q_hs_offset);...
    -l_offset.*sin(q_hf-q_hf_offset)+l1.*cos(q_hf-q_hf_offset).*cos(q_hs+q_hs_offset)+l3.*cos(q_hf-q_hf_offset).*cos(q_hs+q_hs_offset)-l2.*cos(q_hf-q_hf_offset).*cos(q_hs+q_hs_offset).*cos(q_k+q_k_offset)+l2.*cos(q_hf-q_hf_offset).*sin(q_hs+q_hs_offset).*sin(q_k+q_k_offset);...
    l_offset.*cos(q_hf-q_hf_offset)+l1.*sin(q_hf-q_hf_offset).*cos(q_hs+q_hs_offset)+l3.*sin(q_hf-q_hf_offset).*cos(q_hs+q_hs_offset)-l2.*sin(q_hf-q_hf_offset).*cos(q_hs+q_hs_offset).*cos(q_k+q_k_offset)+l2.*sin(q_hf-q_hf_offset).*sin(q_hs+q_hs_offset).*sin(q_k+q_k_offset)];

end

== matlab function husky_sim/Foot placement/Gait timing/Dynamic gait ==
  data: t input; t_start input; y output; T_f input; Ts parameter
% Generate symmetric triangle waves, with amplitude fixed at 1
%
% Input: t_in = clock time;
%       T_f = desired time to peak
%
% Output: triangle wave
function y = func_triangle_wave(t, t_start, T_f, Ts)

% The general triangle wave formula is used:  
%   y = -2*A/p*abs(mod(t,p)-p/2) + A;
%

time = t - t_start;

% Period
p = T_f*2;
% Amplitude, the same as T_f, so the slope is 1
A = T_f;

y = -2*A/p*abs(mod(time,p)-p/2) + A - Ts;

end

== matlab function husky_sim/Foot placement/Gait timing/Transition gait ==
  data: t input; y output; t_start input; T_f input; Ts parameter
% Ramp with upper timit, used to create a timing for a trajectory that
% moves from point A to B only once and stops at point B
%
% Inputs: t - clock time,
%       t_start -  time at which start command is given (from sample and
%           hold)
%       T_f - length of time for trajectory 
%       T_s (param) sample time of system
%
% Output: y = x (ramp starting at 0) with slope of 1 until T_f is reached, 
%        then it saturates at T_f
%       This is because the cubic trajectory os only defined from 0 to T_f
%
function y = func_saturated_ramp(t,t_start,T_f, Ts)

% subtracting Ts because the delay in sample and hold adds 1 Ts to time,
% the multiplier of 0.01 ensure zero crossover to activate rising trigger
time = t - t_start - Ts*1.01;

if time < T_f
    y = time;
else 
    y = T_f;
end
    
end

== matlab function husky_sim/Foot placement/Gait timing/check_transition_end_reached ==
  data: reset_start_time input; y output; switch_to_dynamic input; T_f input; gait_timing input
% Check if end of transition trajectory reached, then reset p0 to current
% reading based off of FK, does not reset for dynamic
%   This ensures, there is no jump in position as start (p0) and end (pf)
%   of trajecotry are the same.
%
% Inputs: reset_start_time: 0 to reset, 1 to start chosen trajectory
%       switch_dynamic: 0 for trasition gait (one shot p0 to pf trajectory)
%                       1 for dynamic (back and forth between two points)
%       T_f: Time taken to reach end of trajecotry
%       gait_timing: timing of chosen trajectory
%
%   Output: 0 of gait not reached, 1 if reached, this activates a rising
%   sample and hold trigger
%
function y = fcn(reset_start_time, switch_to_dynamic, T_f, gait_timing)

if reset_start_time >=1 && switch_to_dynamic == 0 && gait_timing >= T_f 
    y = 1;
else
    y = 0;
end

end

== stateflow chart husky_sim/Foot placement/Chart1 ==
  state Start
    del_p = zeros(1,12);
    T_f = T_f_back_BR;
    reset_start_timer = 0;
    update_p0 = 0;
    p0_out = p_init;
    start_optimizer = 0;
    event = 1;
    count = 0;
    sign_change = 1;
    switch_to_dynamic = 0;
  state Dynamic_FL
    % reset_start_timer = 0;
    update_p0 = 0;
    del_p = [0,0,0, del_p_FL_2, 0,0,0, 0,0,0];
    p0_out = p0_out + del_p;
    v0 = [0,0,0, 0,0,0, 0,0,0, 0,0,0]
    vf = [0,0,0, 0,0,0, 0,0,0, 0,0,0]
    T_f = T_f_FL_2;
    start_optimizer = 1;
    reset_start_timer = 0;
  state Select_event
    % Choose between BR,BL,FL trajectories
    if (count >= n)
    event = event + 1;
    count = 0;
    sign_change = 1;
    end
    if (count >= n/2)
    sign_change = -1;
    end
  state Update_p0_reading
    reset_start_timer = 1;
  state start_dynamic
    reset_start_timer = 1;
    switch_to_dynamic = 1;
  state switch_off
  state Read_p0_encoder
    del_p = zeros(1,12);
    update_p0 = 1;
    reset_start_timer = 0;
  state wait
  state wait1
  state start_move
    reset_start_timer = 1;
  state init_move_BR
    del_p = [0,0,0, 0,0,0, 0,-del_y_BR,del_z_BR(count+1), 0,0,0];
    p0_out = p0_out + del_p;
    if count == 0
    v0 = [0,0,0, 0,0,0, 0,0,0, 0,0,0];
    else
    v0 = [0,0,0, 0,0,0, 0,v_y,v_z, 0,0,0]
    end
    %
    if count == n - 1
    vf = [0,0,0, 0,0,0, 0,0,0, 0,0,0];
    else
    vf = [0,0,0, 0,0,0, 0,v_y,v_z, 0,0,0]
    end
    T_f = T_f_back_BR;
    count = count + 1;
    start_optimizer = 0;
    reset_start_timer = 0;
    update_p0 = 0;
  state init_move_FL
    del_p = [0,0,0, del_p_FL_1, 0,0,0, 0,0,0];
    p0_out = p0_out + del_p;
    v0 = [0,0,0, 0,0,0, 0,0,0, 0,0,0]
    vf = [0,0,0, 0,0,0, 0,0,0, 0,0,0]
    T_f = T_f_FL_1;
    start_optimizer = 1;
    reset_start_timer = 0;
    update_p0 = 0;
    count = n;
  state init_move_BL
    del_p = [0,0,0, 0,0,0, 0,0,0, 0,del_y_BL,del_z_BL(count+1)];
    p0_out = p0_out + del_p;
    %
    if count == 0
    v0 = [0,0,0, 0,0,0, 0,0,0, 0,0,0];
    else
    v0 = [0,0,0, 0,0,0, 0,0,0, 0,v_y,v_z]
    end
    %
    if count == n - 1
    vf = [0,0,0, 0,0,0, 0,0,0, 0,0,0];
    else
    vf = [0,0,0, 0,0,0, 0,0,0, 0,v_y,v_z]
    end
    T_f = T_f_back_BL;
    count = count + 1;
    start_optimizer = 0;
    reset_start_timer = 0;
    update_p0 = 0;
  (default) -> Start
  Start -> Select_event : after(t_start,sec)
  Update_p0_reading -> switch_off
  Select_event -> Dynamic_FL [order 3] : [event == 4]
  Dynamic_FL -> start_dynamic
  switch_off -> Select_event
  Select_event -> init_move_FL [order 1] : [event == 3  && count ~= 0]
  Read_p0_encoder -> Update_p0_reading : after(Ts,sec)
  Select_event -> init_move_BR [order 2] : [event == 1]
  Select_event -> init_move_BL [order 4] : [event == 2 && count ~= 0]
  Select_event -> wait [order 5] : [count == 0 && event > 1]
  start_move -> Read_p0_encoder : after(T_f,sec)
  wait -> wait1 : after(0.2,sec)
  wait1 -> init_move_BL [order 2] : [event == 2]
  wait1 -> init_move_FL [order 1] : [event == 3]
  init_move_BR -> start_move : after(Ts,sec)
  init_move_FL -> start_move : after(Ts,sec)
  init_move_BL -> start_move : after(Ts,sec)
  data: t input; T_f output; del_p output; reset_start_timer output; start_optimizer output; Ts parameter; update_p0 output; t_start parameter; event local; count local; n parameter; sign_change local; p0_out output; p_init parameter; v_z parameter; v_y parameter; v0 output; vf output; del_z_BR parameter; del_z_BL parameter; del_y_BR parameter; del_p_FL_1 parameter; del_p_FL_2 parameter; del_y_BL parameter; T_f_FL_1 parameter; T_f_FL_2 parameter; T_f_back_BR parameter; T_f_back_BL parameter; switch_to_dynamic output
